simulink model "Cruise_Controller_continuous_mdl"  (R2026a)
settings: Solver=VariableStepAuto  StopTime=inf
model workspace (MAT data in the model file):
  MinCruiseSpd = 20
libraries: slpidlib x1
settings Model: Creator=irfan  LastModifiedBy=irfan

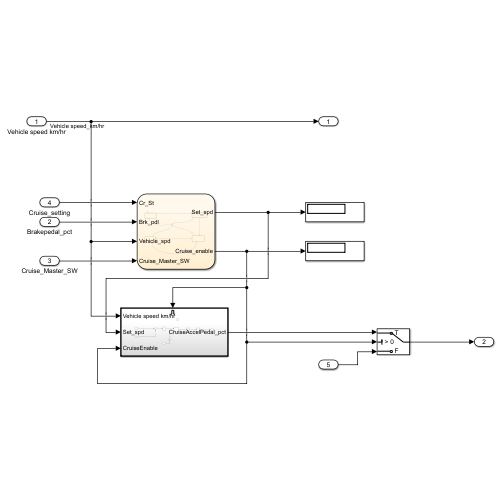
[thumbnail: Simulink's stored preview of the top-level diagram]
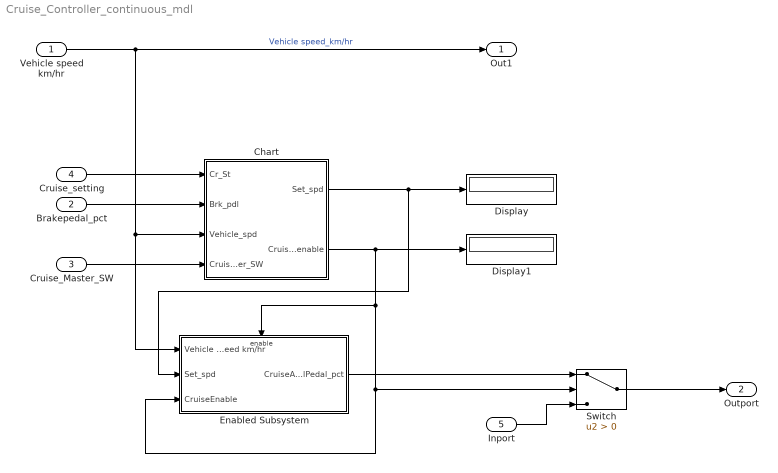
== system Cruise_Controller_continuous_mdl ==
  Vehicle speed km/hr : Inport  OutDataTypeStr=double  PortDimensions=1  SampleTime=0
  Brakepedal_pct : Inport  Port=2  OutDataTypeStr=double  PortDimensions=1
  Cruise_Master_SW : Inport  Port=3  OutDataTypeStr=double  PortDimensions=1
  Cruise_setting : Inport  Port=4  OutDataTypeStr=double  PortDimensions=1
  Inport : Inport  Port=5  OutDataTypeStr=double  PortDimensions=1
  Chart : Stateflow chart  TreatAsAtomicUnit=on
  Display : Display
  Display1 : Display
  Enabled Subsystem : Subsystem  TreatAsAtomicUnit=on
  Switch : Switch  Criteria=u2 > Threshold  SaturateOnIntegerOverflow=off  InputSameDT=off
  Out1 : Outport  OutDataTypeStr=double  PortDimensions=1  SampleTime=0
  Outport : Outport  Port=2  OutDataTypeStr=double  PortDimensions=1
  wires:
  Cruise_setting/1 -> Chart/1(Cr_St)
  Brakepedal_pct/1 -> Chart/2(Brk_pdl)
  Vehicle speed km/hr/1 -> Enabled Subsystem/1(Vehicle speed km/hr), Chart/3(Vehicle_spd), Out1/1  "Vehicle speed_km/hr"
  Chart/1(Set_spd) -> Display/1, Enabled Subsystem/2(Set_spd)
  Chart/2(Cruise_enable) -> Switch/2, Enabled Subsystem/3(CruiseEnable), Enabled Subsystem/Enable, Display1/1
  Cruise_Master_SW/1 -> Chart/4(Cruise_Master_SW)
  Enabled Subsystem/1(CruiseAccelPedal_pct) -> Switch/1
  Inport/1 -> Switch/3
  Switch/1 -> Outport/1

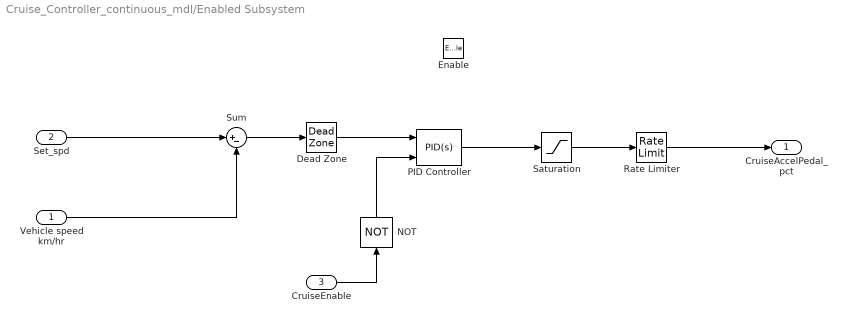
== system Cruise_Controller_continuous_mdl/Enabled Subsystem ==
  Vehicle speed km/hr : Inport
  Set_spd : Inport  Port=2
  CruiseEnable : Inport  Port=3
  Enable : EnablePort  StatesWhenEnabling=reset
  Dead Zone : DeadZone
  NOT : Logic  Operator=NOT  IconShape=distinctive  AllPortsSameDT=off  OutDataTypeStr=boolean
  PID Controller : slpidlib/PID Controller  Controller=PID  Form=Parallel  TimeDomain=Continuous-time  UseExternalTs=off  SampleTime=-1  IntegratorMethod=Forward Euler  FilterMethod=Forward Euler  ControllerParametersSource=internal  P=1  I=0.5  UseKiTs=off  D=0  UseExternalDerivativeSource=off  N=100  UseFilter=on  TunerSelectOption=Transfer Function Based (PID Tuner App)  InitialConditionSource=internal  InitialConditionForIntegrator=0  InitialConditionForFilter=0  DifferentiatorICPrevScaledInput=0  ExternalReset=rising  TrackingMode=off  Kt=1  LimitOutput=on  SatLimitsSource=internal  UpperSaturationLimit=100  LowerSaturationLimit=0  LinearizeAsGain=on  AntiWindupMode=back-calculation  Kb=1  LimitIntegrator=off  UpperIntegratorSaturationLimit=inf  LowerIntegratorSaturationLimit=-inf  POutMin=[]  POutMax=[]  IOutMin=[]  IOutMax=[]  DOutMin=[]  DOutMax=[]  NOutMin=[]  NOutMax=[]  SumOutMin=[]  SumOutMax=[]  SaturationOutMin=[]  SaturationOutMax=[]  PParamMin=[]  PParamMax=[]  IParamMin=[]  IParamMax=[]  DParamMin=[]  DParamMax=[]  NParamMin=[]  NParamMax=[]  KbParamMin=[]  KbParamMax=[]  KtParamMin=[]  KtParamMax=[]  KbOutMin=[]  KbOutMax=[]  KtOutMin=[]  KtOutMax=[]  IntegratorOutMin=[]  IntegratorOutMax=[]  FilterOutMin=[]  FilterOutMax=[]  SumI1OutMin=[]  SumI1OutMax=[]  SumI2OutMin=[]  SumI2OutMax=[]  SumI3OutMin=[]  SumI3OutMax=[]  SumI4OutMin=[]  SumI4OutMax=[]  SumDOutMin=[]  SumDOutMax=[]  DifferentiatorOutMin=[]  DifferentiatorOutMax=[]  FilterDiffOutCoefMin=[]  FilterDiffOutCoefMax=[]  ReciprocalOutMin=[]  ReciprocalOutMax=[]  SumDenOutMin=[]  SumDenOutMax=[]  SumNumOutMin=[]  SumNumOutMax=[]  DivideOutMin=[]  DivideOutMax=[]  UdiffTsProdOutMin=[]  UdiffTsProdOutMax=[]  NTsProdOutMin=[]  NTsProdOutMax=[]  UintegralTsProdOutMin=[]  UintegralTsProdOutMax=[]  UngainTsProdOutMin=[]  UngainTsProdOutMax=[]  ClampingZeroOutDataTypeStr=Inherit: Inherit via back propagation  ClampingZeroOutMin=[]  ClampingZeroOutMax=[]  FilterDenConstantOutDataTypeStr=Inherit: Inherit via back propagation  FilterDenConstantOutMin=[]  FilterDenConstantOutMax=[]  PCopyOutDataTypeStr=Inherit: Inherit via back propagation  PCopyOutMin=[]  PCopyOutMax=[]  NCopyOutDataTypeStr=Inherit: Inherit via back propagation  NCopyOutMin=[]  NCopyOutMax=[]  IntegratorContinuousStateAttributes=''  IntegratorStateMustResolveToSignalObject=off  IntegratorRTWStateStorageClass=Auto  FilterContinuousStateAttributes=''  FilterStateMustResolveToSignalObject=off  FilterRTWStateStorageClass=Auto  ParallelPVariant=InternalParameters  IdealPVariant=Disabled  IVariant=InternalParameters  DVariant=InternalParameters  IntegratorVariant=Continuous  SatVariant=Enabled  AWVariant=BackCalculation  PCopyVariant=Disabled  TRVariant=Disabled  FdbkBlocksVariant=Forward  IdealPFdbkVariant=Disabled  SatFdbkVariant=Disabled  DerivativeFilterVariant=ContFilter  NVariant=InternalParameters  NCopyVariant=Disabled  FilterICVariant=InternalICsFilter  IntegratorICVariant=InternalICs  ExternalResetVariant=ExternalReset  TRSumVariant=Passthrough  SumFdbkVariant=Disabled  SumVariant=Sum_PID  TsampFilterVariant=InternalTs  TsampNgainVariant=Passthrough  TsampIntegralVariant=Disabled_SignalSpec  ExternalSaturationOutDataTypeStr=Inherit: Same as second input  DerivativeSourceVariant=ErrorSignal  PreIntVariant=InternalPreInt
  Rate Limiter : RateLimiter  RisingSlewLimit=25  FallingSlewLimit=-40  SampleTimeMode=inherited
  Saturation : Saturate  UpperLimit=100  LowerLimit=0
  Sum : Sum  Inputs=|+-
  CruiseAccelPedal_pct : Outport
  wires:
  Dead Zone/1 -> PID Controller/1
  Rate Limiter/1 -> CruiseAccelPedal_pct/1
  PID Controller/1 -> Saturation/1
  Set_spd/1 -> Sum/1
  Vehicle speed km/hr/1 -> Sum/2
  NOT/1 -> PID Controller/2
  CruiseEnable/1 -> NOT/1
  Saturation/1 -> Rate Limiter/1
  Sum/1 -> Dead Zone/1

== stateflow chart Cruise_Controller_continuous_mdl/Chart ==
  state READY
    entry:
    Set_spd = Vehicle_spd;
    Cruise_enable=0;
  state OFF
    during:
    Cruise_enable=0;
  state ACTIVE
    during:
    Cruise_enable=1;
  state STANDBY
    during:
    Cruise_enable=0;
  (default) -> OFF
  OFF -> READY : [Cruise_Master_SW==1 && Cr_St==1 && Vehicle_spd>MinCruiseSpd]
  READY -> (junction 19) [order 2]
  READY -> ACTIVE [order 1] : [true]
  (junction 19) -> OFF : [Cruise_Master_SW==0]
  ACTIVE -> (junction 19) [order 2]
  STANDBY -> (junction 19) [order 2]
  ACTIVE -> STANDBY [order 1] : [Cruise_Master_SW==1 && Cr_St==0 || Brk_pdl>0]
  STANDBY -> ACTIVE [order 1] : [Cruise_Master_SW==1 && Cr_St==2]
  data: Cr_St input; Brk_pdl input; Set_spd output; Cruise_enable output; Vehicle_spd input; MinCruiseSpd parameter; Cruise_Master_SW input
